simulink model "w3_warplab_trigger_proc"  (Simulink 7.7)
settings: Solver=ode45  StartTime=0.0  StopTime=60  RelTol=1e-3
InitFcn:
  | w3_warplab_trigger_proc_init
StartFcn:
  | w3_warplab_trigger_proc_init
undefined symbols (not defined in the file): gcbh, xlBlockLoadCallback, xlGetNormalizedPeriod
libraries: xbsIndex_r4 x1289, xbsEDKLib_r4 x1, simulink x1
(part 2 of 10)

== system w3_warplab_trigger_proc/CM-PLL Outputs ==
  note: NOTE:  EXT_OUT_P0 (ie trig_2) should be at bit
      |         position 0 on the trigs_in bus for the Black Box.
  note: NOTE:  Black Box contains a register packed into the IOB for
      |     trigger input.  No need for additional register on this path.
  "trig_2 " : Inport
  "trig_3 " : Inport  Port=2
  "trig_4 " : Inport  Port=3
  "trig_5 " : Inport  Port=4
  Black Box : xbsIndex_r4/Black Box  init_code=trig_odelays_config  sim_method=ISE Simulator  verbose=off  block_type=blackbox2
  Concat : xbsIndex_r4/Concat  num_inputs=4  dbl_ovrd=off  block_type=concat
  Constant : xbsIndex_r4/Constant  const=0  gui_display_data_type=Boolean  arith_type=Boolean  n_bits=16  bin_pt=14  preci_type=Single  exp_width=8  frac_width=24  explicit_period=off  period=1  equ=P=C  opselect=C  inp2=PCIN>>17  opr=+  inp1=P  carry=CIN  dbl_ovrd=off  block_type=constant
  Terminator{1..3,16} (4 alike) : Terminator
  b[0] : xbsIndex_r4/Slice  nbits=1  boolean_output=off  mode=Lower Bit Location + Width  bit1=0  base1=MSB of Input  bit0=0  base0=LSB of Input  dbl_ovrd=off  block_type=slice
  b[1] : xbsIndex_r4/Slice  nbits=1  boolean_output=off  mode=Lower Bit Location + Width  bit1=0  base1=MSB of Input  bit0=1  base0=LSB of Input  dbl_ovrd=off  block_type=slice
  b[2] : xbsIndex_r4/Slice  nbits=1  boolean_output=off  mode=Lower Bit Location + Width  bit1=0  base1=MSB of Input  bit0=2  base0=LSB of Input  dbl_ovrd=off  block_type=slice
  b[3] : xbsIndex_r4/Slice  nbits=1  boolean_output=off  mode=Lower Bit Location + Width  bit1=0  base1=MSB of Input  bit0=3  base0=LSB of Input  dbl_ovrd=off  block_type=slice
  cm_pll_0_out : xbsIndex_r4/Gateway Out  inherit_from_input=off  hdl_port=on  timing_constraint=None  locs_specified=off  LOCs={}  UseAsDAC=off  DACChannel='1'  block_type=gatewayout
  cm_pll_1_out : xbsIndex_r4/Gateway Out  inherit_from_input=off  hdl_port=on  timing_constraint=None  locs_specified=off  LOCs={}  UseAsDAC=off  DACChannel='1'  block_type=gatewayout
  cm_pll_2_out : xbsIndex_r4/Gateway Out  inherit_from_input=off  hdl_port=on  timing_constraint=None  locs_specified=off  LOCs={}  UseAsDAC=off  DACChannel='1'  block_type=gatewayout
  cm_pll_3_out : xbsIndex_r4/Gateway Out  inherit_from_input=off  hdl_port=on  timing_constraint=None  locs_specified=off  LOCs={}  UseAsDAC=off  DACChannel='1'  block_type=gatewayout
  wires:
  b[0]/1 -> cm_pll_0_out/1
  b[1]/1 -> cm_pll_1_out/1
  b[2]/1 -> cm_pll_2_out/1
  b[3]/1 -> cm_pll_3_out/1
  Black Box/1 -> b[0]/1, b[1]/1, b[2]/1, b[3]/1
  cm_pll_0_out/1 -> Terminator16/1
  cm_pll_1_out/1 -> Terminator1/1
  cm_pll_2_out/1 -> Terminator2/1
  cm_pll_3_out/1 -> Terminator3/1
  "trig_2 "/1 -> Concat/4
  "trig_3 "/1 -> Concat/3
  "trig_4 "/1 -> Concat/2
  "trig_5 "/1 -> Concat/1
  Constant/1 -> Black Box/1
  Concat/1 -> Black Box/2
  [TRIG_OUT_ODELAY_CMPLL0] -> Black Box/3
  [TRIG_OUT_ODELAY_CMPLL1] -> Black Box/4
  [TRIG_OUT_ODELAY_CMPLL2] -> Black Box/5
  [TRIG_OUT_ODELAY_CMPLL3] -> Black Box/6
  [TRIG_OUT_ODELAYS_UPDATE] -> Black Box/7

== system w3_warplab_trigger_proc/Debug Header Outputs 1 ==
  note: NOTE:  EXT_OUT_P0 (ie trig_2) should be at bit
      |         position 0 on the trigs_in bus for the Black Box.
  note: NOTE:  Black Box contains a register packed into the IOB for
      |     trigger input.  No need for additional register on this path.
  "trig_2 " : Inport
  "trig_3 " : Inport  Port=2
  "trig_4 " : Inport  Port=3
  "trig_5 " : Inport  Port=4
  Black Box : xbsIndex_r4/Black Box  init_code=trig_odelays_config  sim_method=ISE Simulator  verbose=off  block_type=blackbox2
  Concat : xbsIndex_r4/Concat  num_inputs=4  dbl_ovrd=off  block_type=concat
  Constant : xbsIndex_r4/Constant  const=0  gui_display_data_type=Boolean  arith_type=Boolean  n_bits=16  bin_pt=14  preci_type=Single  exp_width=8  frac_width=24  explicit_period=off  period=1  equ=P=C  opselect=C  inp2=PCIN>>17  opr=+  inp1=P  carry=CIN  dbl_ovrd=off  block_type=constant
  b[0] : xbsIndex_r4/Slice  nbits=1  boolean_output=off  mode=Lower Bit Location + Width  bit1=0  base1=MSB of Input  bit0=0  base0=LSB of Input  dbl_ovrd=off  block_type=slice
  b[1] : xbsIndex_r4/Slice  nbits=1  boolean_output=off  mode=Lower Bit Location + Width  bit1=0  base1=MSB of Input  bit0=1  base0=LSB of Input  dbl_ovrd=off  block_type=slice
  b[2] : xbsIndex_r4/Slice  nbits=1  boolean_output=off  mode=Lower Bit Location + Width  bit1=0  base1=MSB of Input  bit0=2  base0=LSB of Input  dbl_ovrd=off  block_type=slice
  b[3] : xbsIndex_r4/Slice  nbits=1  boolean_output=off  mode=Lower Bit Location + Width  bit1=0  base1=MSB of Input  bit0=3  base0=LSB of Input  dbl_ovrd=off  block_type=slice
  trig_2_0_out : xbsIndex_r4/Gateway Out  inherit_from_input=off  hdl_port=on  timing_constraint=None  locs_specified=off  LOCs={}  UseAsDAC=off  DACChannel='1'  block_type=gatewayout
  trig_3_0_out : xbsIndex_r4/Gateway Out  inherit_from_input=off  hdl_port=on  timing_constraint=None  locs_specified=off  LOCs={}  UseAsDAC=off  DACChannel='1'  block_type=gatewayout
  trig_4_0_out : xbsIndex_r4/Gateway Out  inherit_from_input=off  hdl_port=on  timing_constraint=None  locs_specified=off  LOCs={}  UseAsDAC=off  DACChannel='1'  block_type=gatewayout
  trig_5_0_out : xbsIndex_r4/Gateway Out  inherit_from_input=off  hdl_port=on  timing_constraint=None  locs_specified=off  LOCs={}  UseAsDAC=off  DACChannel='1'  block_type=gatewayout
  trig_2 : Outport
  trig_3 : Outport  Port=2
  trig_4 : Outport  Port=3
  trig_5 : Outport  Port=4
  wires:
  b[0]/1 -> trig_2_0_out/1
  b[1]/1 -> trig_3_0_out/1
  b[2]/1 -> trig_4_0_out/1
  b[3]/1 -> trig_5_0_out/1
  Black Box/1 -> b[0]/1, b[1]/1, b[2]/1, b[3]/1
  trig_2_0_out/1 -> trig_2/1  "Out 2"
  trig_3_0_out/1 -> trig_3/1  "Out 3"
  trig_4_0_out/1 -> trig_4/1  "Out 4"
  trig_5_0_out/1 -> trig_5/1  "Out 5"
  "trig_2 "/1 -> Concat/4
  "trig_3 "/1 -> Concat/3
  "trig_4 "/1 -> Concat/2
  "trig_5 "/1 -> Concat/1
  Constant/1 -> Black Box/1
  Concat/1 -> Black Box/2
  [TRIG_OUT_ODELAY_DBG0] -> Black Box/3
  [TRIG_OUT_ODELAY_DBG1] -> Black Box/4
  [TRIG_OUT_ODELAY_DBG2] -> Black Box/5
  [TRIG_OUT_ODELAY_DBG3] -> Black Box/6
  [TRIG_OUT_ODELAYS_UPDATE] -> Black Box/7

== system w3_warplab_trigger_proc/Debug Header Outputs 2 ==
  note: NOTE:  EXT_OUT_P0 (ie trig_2) should be at bit
      |         position 0 on the trigs_in bus for the Black Box.
  note: NOTE:  Black Box contains a register packed into the IOB for
      |     trigger input.  No need for additional register on this path.
  "trig_2 " : Inport
  "trig_3 " : Inport  Port=2
  "trig_4 " : Inport  Port=3
  "trig_5 " : Inport  Port=4
  Black Box : xbsIndex_r4/Black Box  init_code=trig_odelays_config  sim_method=ISE Simulator  verbose=off  block_type=blackbox2
  Concat : xbsIndex_r4/Concat  num_inputs=4  dbl_ovrd=off  block_type=concat
  Constant : xbsIndex_r4/Constant  const=0  gui_display_data_type=Boolean  arith_type=Boolean  n_bits=16  bin_pt=14  preci_type=Single  exp_width=8  frac_width=24  explicit_period=off  period=1  equ=P=C  opselect=C  inp2=PCIN>>17  opr=+  inp1=P  carry=CIN  dbl_ovrd=off  block_type=constant
  Terminator{1..3,16} (4 alike) : Terminator
  b[0] : xbsIndex_r4/Slice  nbits=1  boolean_output=off  mode=Lower Bit Location + Width  bit1=0  base1=MSB of Input  bit0=0  base0=LSB of Input  dbl_ovrd=off  block_type=slice
  b[1] : xbsIndex_r4/Slice  nbits=1  boolean_output=off  mode=Lower Bit Location + Width  bit1=0  base1=MSB of Input  bit0=1  base0=LSB of Input  dbl_ovrd=off  block_type=slice
  b[2] : xbsIndex_r4/Slice  nbits=1  boolean_output=off  mode=Lower Bit Location + Width  bit1=0  base1=MSB of Input  bit0=2  base0=LSB of Input  dbl_ovrd=off  block_type=slice
  b[3] : xbsIndex_r4/Slice  nbits=1  boolean_output=off  mode=Lower Bit Location + Width  bit1=0  base1=MSB of Input  bit0=3  base0=LSB of Input  dbl_ovrd=off  block_type=slice
  trig_2_1_out : xbsIndex_r4/Gateway Out  inherit_from_input=off  hdl_port=on  timing_constraint=None  locs_specified=off  LOCs={}  UseAsDAC=off  DACChannel='1'  block_type=gatewayout
  trig_3_1_out : xbsIndex_r4/Gateway Out  inherit_from_input=off  hdl_port=on  timing_constraint=None  locs_specified=off  LOCs={}  UseAsDAC=off  DACChannel='1'  block_type=gatewayout
  trig_4_1_out : xbsIndex_r4/Gateway Out  inherit_from_input=off  hdl_port=on  timing_constraint=None  locs_specified=off  LOCs={}  UseAsDAC=off  DACChannel='1'  block_type=gatewayout
  trig_5_1_out : xbsIndex_r4/Gateway Out  inherit_from_input=off  hdl_port=on  timing_constraint=None  locs_specified=off  LOCs={}  UseAsDAC=off  DACChannel='1'  block_type=gatewayout
  wires:
  Black Box/1 -> b[3]/1, b[2]/1, b[1]/1, b[0]/1
  b[3]/1 -> trig_5_1_out/1
  b[2]/1 -> trig_4_1_out/1
  b[1]/1 -> trig_3_1_out/1
  b[0]/1 -> trig_2_1_out/1
  trig_2_1_out/1 -> Terminator16/1
  trig_3_1_out/1 -> Terminator1/1
  trig_4_1_out/1 -> Terminator2/1
  trig_5_1_out/1 -> Terminator3/1
  "trig_2 "/1 -> Concat/4
  "trig_3 "/1 -> Concat/3
  "trig_4 "/1 -> Concat/2
  "trig_5 "/1 -> Concat/1
  Constant/1 -> Black Box/1
  Concat/1 -> Black Box/2
  [TRIG_OUT_ODELAY_DBG0] -> Black Box/3
  [TRIG_OUT_ODELAY_DBG1] -> Black Box/4
  [TRIG_OUT_ODELAY_DBG2] -> Black Box/5
  [TRIG_OUT_ODELAY_DBG3] -> Black Box/6
  [TRIG_OUT_ODELAYS_UPDATE] -> Black Box/7
